simulink model "DevelopmentModel"  (R2014b)
settings: Solver=ode45  StartTime=0.0  StopTime=120  FixedStep=0.05  RelTol=1e-3
libraries: LegIK x6, MainController x1, TestSequence x1, Coord_BodyToLeg x1, TriggerSystem x1, Completemodels x1
settings Model: Creator=Sebastian  LastModifiedBy=Sebastian
settings DataIOCC: SaveOutput=off  OutputOption=SpecifiedOutputTimes  OutputTimes=[0:1/30:120]
settings OptimizationCC: ZeroExternalMemoryAtStartup=off  ZeroInternalMemoryAtStartup=off  NoFixptDivByZeroProtection=on  EfficientFloat2IntCast=on  OptimizeModelRefInitCode=on  LifeSpan=1
settings DebuggingCC: BusObjectLabelMismatch=error  AssertControl=DisableAll
settings HardwareCC: ProdBitPerInt=16  ProdBitPerPointer=8  ProdIntDivRoundTo=Zero  ProdEndianess=LittleEndian  ProdWordSize=8  ProdHWDeviceType=Atmel->AVR
settings RTWCC: SystemTargetFile=arduino_ec.tlc  TemplateMakefile=arduino_ec.tmf  Description=Arduino EC Target  GenerateReport=on  ProcessScript=arduino_ec_make_rtw_hook  IncludeHyperlinkInReport=on  LaunchReport=on
settings CodeAppCC: IgnoreCustomStorageClasses=off
settings STFCustomTargetCC: TargetLibSuffix=.a  UtilityFuncGeneration=Shared location  GenerateSampleERTMain=on  CombineOutputUpdateFcns=on  ERTCustomFileBanners=on  SupportNonFinite=off  SupportContinuousTime=off  SupportNonInlinedSFcns=off  ParenthesesLevel=Maximum  CastingMode=Standards  MATLABClassNameForMDSCustomization=Simulink.SoftwareTarget.ERTCustomization  GRTInterface=off  GenerateSharedConstants=off  SystemTargetFile=arduino_ec.tlc
settings ERTTargetCC: UtilityFuncGeneration=Shared location  GenerateSampleERTMain=on  ParMdlRefBuildCompliant=off  CompOptLevelCompliant=off  ConcurrentExecutionCompliant=off  ERTFirstTimeCompliant=off  SupportNonFinite=off  ParenthesesLevel=Maximum  CastingMode=Standards  ModelStepFunctionPrototypeControlCompliant=off  CPPClassGenCompliant=off  GenerateSharedConstants=off  InlinedParameterPlacement=NonHierarchical  ERTCustomFileTemplate=arduino_ec_file_process.tlc

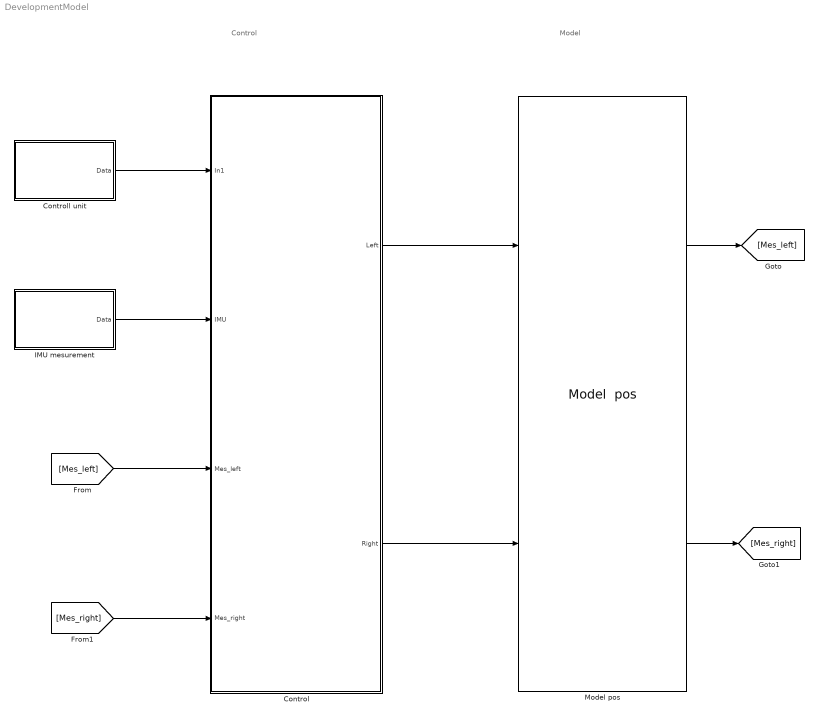
== system DevelopmentModel ==
  note: Model
  note: Control
  Control : Subsystem  TreatAsAtomicUnit=on
  Controll unit : Subsystem
  IMU mesurement : Subsystem
  Model pos : Completemodels/Model  pos
  wires:
  IMU mesurement/1(Data) -> Control/2(IMU)
  Model pos/1 -> [Mes_left]
  Control/1(Left) -> Model pos/1
  Control/2(Right) -> Model pos/2
  Model pos/2 -> [Mes_right]
  [Mes_right] -> Control/4(Mes_right)
  [Mes_left] -> Control/3(Mes_left)
  Controll unit/1(Data) -> Control/1(In1)

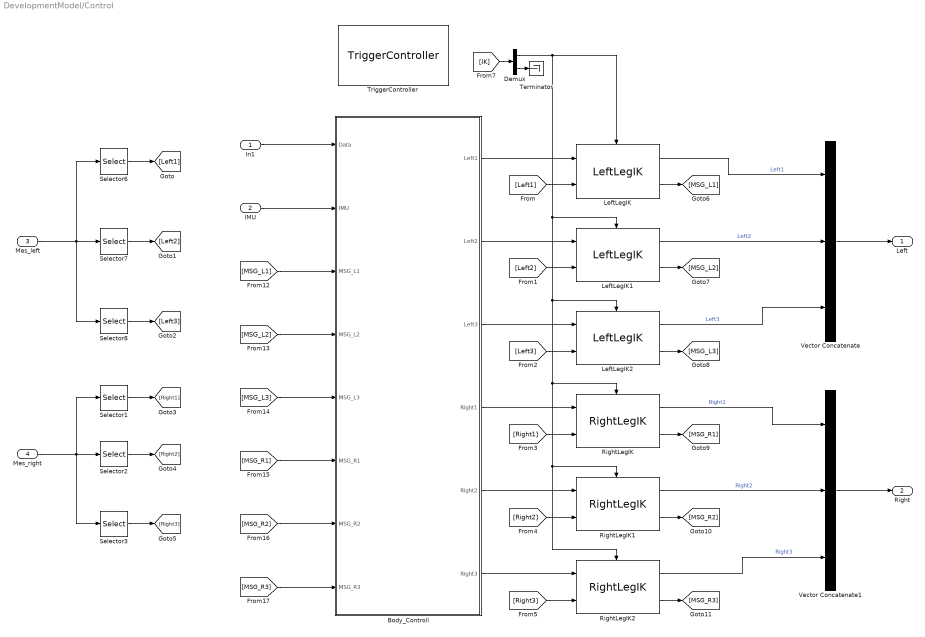
== system DevelopmentModel/Control ==
  In1 : Inport
  IMU : Inport  Port=2
  Mes_left : Inport  Port=3  OutDataTypeStr=Bus: Leg_mes
  Mes_right : Inport  Port=4  OutDataTypeStr=Bus: Leg_mes
  Body_Controll : Subsystem
  Demux : Demux  Outputs=2
  LeftLegIK : LegIK/LeftLegIK  ID1=1  ID2=3  ID3=5
  LeftLegIK1 : LegIK/LeftLegIK  ID1=13  ID2=15  ID3=17
  LeftLegIK2 : LegIK/LeftLegIK  ID1=7  ID2=9  ID3=11
  RightLegIK : LegIK/RightLegIK  ID1=2  ID2=4  ID3=6
  RightLegIK1 : LegIK/RightLegIK  ID1=14  ID2=16  ID3=18
  RightLegIK2 : LegIK/RightLegIK  ID1=8  ID2=10  ID3=12
  Selector1 : Selector  IndexMode=Zero-based  InputPortWidth=3  Indices=0
  Selector2 : Selector  IndexMode=Zero-based  InputPortWidth=3
  Selector3 : Selector  IndexMode=Zero-based  InputPortWidth=3  Indices=2
  Selector6 : Selector  IndexMode=Zero-based  InputPortWidth=3  Indices=0
  Selector7 : Selector  IndexMode=Zero-based  InputPortWidth=3
  Selector8 : Selector  IndexMode=Zero-based  InputPortWidth=3  Indices=2
  Terminator : Terminator
  TriggerController : TriggerSystem/TriggerController  f=40
  Vector Concatenate : Concatenate  NumInputs=3  ConcatenateDimension=2
  Vector Concatenate1 : Concatenate  NumInputs=3  ConcatenateDimension=2
  Left : Outport  OutDataTypeStr=Bus: Leg_ref
  Right : Outport  Port=2  OutDataTypeStr=Bus: Leg_ref
  wires:
  Body_Controll/2(Left2) -> LeftLegIK1/1
  Body_Controll/1(Left1) -> LeftLegIK/1
  Body_Controll/3(Left3) -> LeftLegIK2/1
  Body_Controll/5(Right2) -> RightLegIK1/1
  Body_Controll/4(Right1) -> RightLegIK/1
  Body_Controll/6(Right3) -> RightLegIK2/1
  In1/1 -> Body_Controll/1(Data)
  [Left3] -> LeftLegIK2/2
  [Right1] -> RightLegIK/2
  RightLegIK/2 -> [MSG_R1]
  [MSG_R3] -> Body_Controll/8(MSG_R3)
  [MSG_R2] -> Body_Controll/7(MSG_R2)
  [MSG_R1] -> Body_Controll/6(MSG_R1)
  [MSG_L3] -> Body_Controll/5(MSG_L3)
  [MSG_L2] -> Body_Controll/4(MSG_L2)
  [MSG_L1] -> Body_Controll/3(MSG_L1)
  RightLegIK2/2 -> [MSG_R3]
  LeftLegIK2/2 -> [MSG_L3]
  RightLegIK1/2 -> [MSG_R2]
  LeftLegIK1/2 -> [MSG_L2]
  LeftLegIK/2 -> [MSG_L1]
  [Right2] -> RightLegIK1/2
  IMU/1 -> Body_Controll/2(IMU)
  [Right3] -> RightLegIK2/2
  [Left1] -> LeftLegIK/2
  [Left2] -> LeftLegIK1/2
  LeftLegIK2/1 -> Vector Concatenate/3  "Left3"
  LeftLegIK1/1 -> Vector Concatenate/2  "Left2"
  LeftLegIK/1 -> Vector Concatenate/1  "Left1"
  Vector Concatenate/1 -> Left/1
  RightLegIK/1 -> Vector Concatenate1/1  "Right1"
  RightLegIK1/1 -> Vector Concatenate1/2  "Right2"
  RightLegIK2/1 -> Vector Concatenate1/3  "Right3"
  Vector Concatenate1/1 -> Right/1
  Mes_left/1 -> Selector6/1, Selector7/1, Selector8/1
  Selector6/1 -> [Left1]
  Selector7/1 -> [Left2]
  Selector8/1 -> [Left3]
  Mes_right/1 -> Selector3/1, Selector2/1, Selector1/1
  Selector1/1 -> [Right1]
  Selector2/1 -> [Right2]
  Selector3/1 -> [Right3]
  Demux/1 -> RightLegIK1/Trigger, RightLegIK2/Trigger, RightLegIK/Trigger, LeftLegIK2/Trigger, LeftLegIK1/Trigger, LeftLegIK/Trigger
  [IK] -> Demux/1
  Demux/2 -> Terminator/1

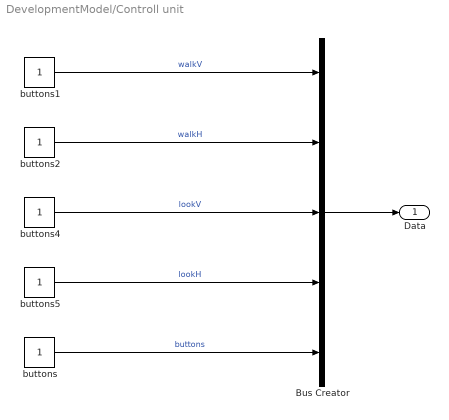
== system DevelopmentModel/Controll unit ==
  Bus Creator : BusCreator  Inputs=5  OutDataTypeStr=Bus: Command
  buttons : Constant  OutDataTypeStr=uint8
  buttons{1..2,4..5} (4 alike) : Constant  OutDataTypeStr=int8
  Data : Outport  OutDataTypeStr=Bus: Command  PortDimensions=3
  wires:
  buttons/1 -> Bus Creator/5  "buttons"
  buttons1/1 -> Bus Creator/1  "walkV"
  buttons2/1 -> Bus Creator/2  "walkH"
  buttons4/1 -> Bus Creator/3  "lookV"
  buttons5/1 -> Bus Creator/4  "lookH"
  Bus Creator/1 -> Data/1

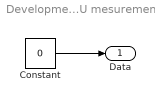
== system DevelopmentModel/IMU mesurement ==
  Constant : Constant  Value=0  OutDataTypeStr=int8
  Data : Outport
  wires:
  Constant/1 -> Data/1

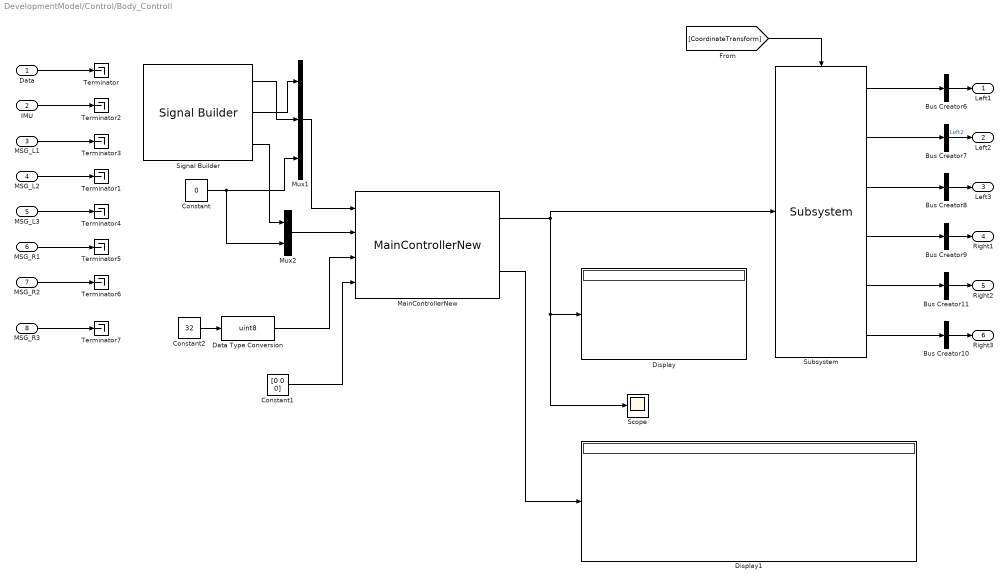
== system DevelopmentModel/Control/Body_Controll ==
  Data : Inport  OutDataTypeStr=Bus: Command
  IMU : Inport  Port=2  OutDataTypeStr=int8
  MSG_L1 : Inport  Port=3
  MSG_L2 : Inport  Port=4
  MSG_L3 : Inport  Port=5
  MSG_R1 : Inport  Port=6
  MSG_R2 : Inport  Port=7
  MSG_R3 : Inport  Port=8
  Bus Creator{6..11} (6 alike) : BusCreator  Inputs=1  OutDataTypeStr=Bus: Leg_data
      settings: InheritFromInputs=off
  Constant : Constant  Value=0
  Constant1 : Constant  Value=[0 0 0]
  Constant2 : Constant  Value=32
  Data Type Conversion : DataTypeConversion  OutDataTypeStr=uint8
  Display : Display
  Display1 : Display
  MainControllerNew : MainController/MainControllerNew
  Mux1 : Mux  Inputs=3
  Mux2 : Mux  Inputs=2
  Scope : Scope
      settings: YMin=-250  YMax=250  SaveName=ScopeData5
  Signal Builder : TestSequence/TestSequence/Signal Builder  Tag=STV Subsys
  Subsystem : Coord_BodyToLeg/Subsystem
  Terminator{,1..7} (8 alike) : Terminator
  Left1 : Outport  OutDataTypeStr=Bus: Leg_data
  Left2 : Outport  Port=2  OutDataTypeStr=Bus: Leg_data
  Left3 : Outport  Port=3  OutDataTypeStr=Bus: Leg_data
  Right1 : Outport  Port=4  OutDataTypeStr=Bus: Leg_data
  Right2 : Outport  Port=5  OutDataTypeStr=Bus: Leg_data
  Right3 : Outport  Port=6  OutDataTypeStr=Bus: Leg_data
  wires:
  Data/1 -> Terminator/1
  MSG_R3/1 -> Terminator7/1
  IMU/1 -> Terminator2/1
  MSG_L1/1 -> Terminator3/1
  MSG_L2/1 -> Terminator1/1
  MSG_L3/1 -> Terminator4/1
  MSG_R1/1 -> Terminator5/1
  MSG_R2/1 -> Terminator6/1
  Subsystem/1 -> Bus Creator6/1
  Subsystem/2 -> Bus Creator7/1
  Subsystem/3 -> Bus Creator8/1
  Subsystem/4 -> Bus Creator9/1
  Subsystem/5 -> Bus Creator11/1
  Subsystem/6 -> Bus Creator10/1
  Bus Creator10/1 -> Right3/1
  Bus Creator11/1 -> Right2/1
  Bus Creator9/1 -> Right1/1
  Bus Creator8/1 -> Left3/1
  Bus Creator7/1 -> Left2/1  "Left2"
  Bus Creator6/1 -> Left1/1
  Mux1/1 -> MainControllerNew/1
  MainControllerNew/1 -> Scope/1, Display/1, Subsystem/1
  MainControllerNew/2 -> Display1/1
  Constant2/1 -> Data Type Conversion/1
  Data Type Conversion/1 -> MainControllerNew/3
  Constant1/1 -> MainControllerNew/4
  [CoordinateTransform] -> Subsystem/Trigger
  Mux2/1 -> MainControllerNew/2
  Signal Builder/3 -> Mux2/1
  Constant/1 -> Mux2/2, Mux1/3
  Signal Builder/1 -> Mux1/2
  Signal Builder/2 -> Mux1/1
